simulink model "traffic"  (R2017a)
settings: Solver=ode45  StartTime=0.0  StopTime=30.0  RelTol=1e-3  EnableMultiTasking=on
undefined symbols (not defined in the file): des, gcbh
settings Model: Creator=pathmapirian  LastModifiedBy=PRAGA SV
settings DataIOCC: LimitDataPoints=on  SaveFormat=Array
settings OptimizationCC: LifeSpan=inf
settings DebuggingCC: UnderspecifiedInitializationDetection=Classic  MergeDetectMultiDrivingBlocksExec=none  SolverPrmCheckMsg=warning  StateNameClashWarn=warning  SFUnexpectedBacktrackingDiag=warning  SFNoUnconditionalDefaultTransitionDiag=warning  SFExecutionAtInitializationDiag=none
settings HardwareCC: ProdBitPerPointer=32  ProdBitPerSizeT=32  ProdBitPerPtrDiffT=32  ProdLargestAtomicFloat=None  ProdIntDivRoundTo=Undefined  ProdEndianess=Unspecified  ProdWordSize=32  ProdHWDeviceType=32-bit Generic
settings ModelReferenceCC: PropagateSignalLabelsOutOfModel=off
settings GRTTargetCC: TargetLangStandard=C89/C90 (ANSI)  GeneratePreprocessorConditionals=Disable all
settings ConfigComp: CovMetricSettings=dw  CovHtmlReporting=on  CovSaveCumulativeToWorkspaceVar=on  CovSaveSingleToWorkspaceVar=on  CovExternalEMLEnable=off

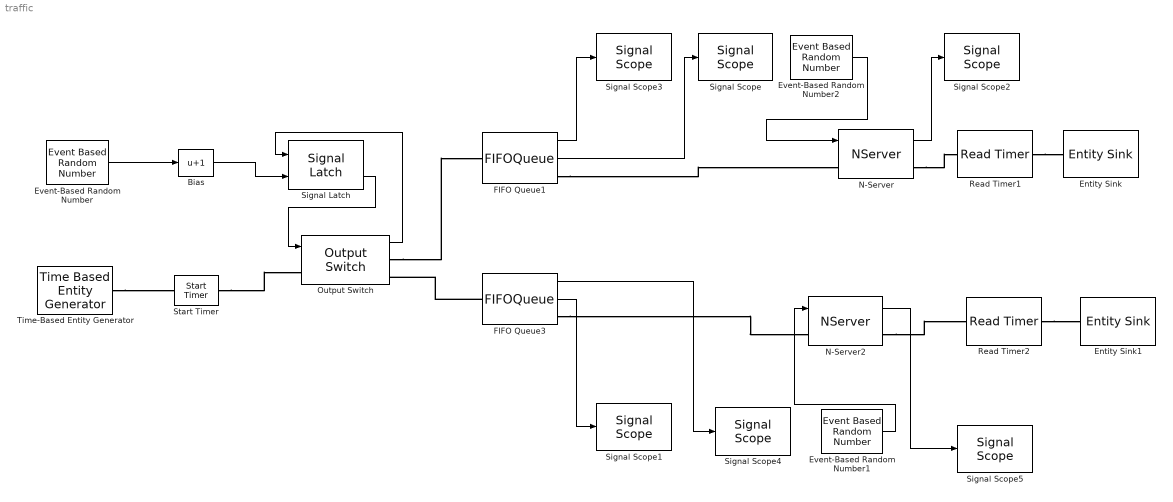
== system traffic ==
  Bias : Bias  Bias=1
  Entity Sink : EntitySink
  Entity Sink1 : EntitySink
  Event-Based Random Number : EventBasedRandomNumber  Distribution=Bernoulli  pOneBern=0.6  Seed=10
  Event-Based Random Number1 : EventBasedRandomNumber  Distribution=Uniform
  Event-Based Random Number2 : EventBasedRandomNumber
  FIFO Queue1 : FIFOQueue  StatNumberInBlock=on  StatAverageWait=on
      settings: OutputPortMap=o1,o2
  FIFO Queue3 : FIFOQueue  StatNumberInBlock=on  StatAverageWait=on
      settings: OutputPortMap=o1,o2
  N-Server : NServer  NumberOfServers=1  ServiceTimeFrom=Signal port t  StatUtilization=on
      settings: OutputPortMap=o5
  N-Server2 : NServer  NumberOfServers=1  ServiceTimeFrom=Signal port t  StatUtilization=on
      settings: OutputPortMap=o5
  Output Switch : OutputSwitch  NumberOutputPorts=2  SwitchingCriterion=From signal port p  InitialConditionsOpt=on  StatNumberDeparted=on
  Read Timer1 : ReadTimer
  Read Timer2 : ReadTimer
  Signal Latch : SignalLatch  ReadMemoryUpon=Write to memory event  ReportMemoryUponWrite=on
      settings: InputPortMap=u0,u2  OutputPortMap=o1,o2
  Signal Scope{,1..5} (6 alike) : SignalScope  LoadFcn=des.scope.CallbackSupport('seLoadFcn',gcbh)  StartFcn=des.scope.CallbackSupport('seStartFcn',gcbh)  StopFcn=des.scope.CallbackSupport('seStopFcn',gcbh)
      settings: CopyFcn=des.scope.CallbackSupport('seCopyFcn',gcbh)  DeleteFcn=des.scope.CallbackSupport('seDeleteFcn',gcbh)  PreSaveFcn=des.scope.CallbackSupport('sePreSaveFcn',gcbh)  NameChangeFcn=des.scope.CallbackSupport('seNameChangeFcn',gcbh)  OpenFcn=des.scope.CallbackSupport('seOpenFcn',gcbh)
  Start Timer : StartTimer
  Time-Based Entity Generator : TimeBasedEntityGenerator
  wires:
  FIFO Queue1/1 -> Signal Scope3/1
  FIFO Queue1/2 -> Signal Scope/1
  Event-Based Random Number2/1 -> N-Server/1
  N-Server/1 -> Signal Scope2/1
  FIFO Queue3/2 -> Signal Scope1/1
  FIFO Queue3/1 -> Signal Scope4/1
  Event-Based Random Number1/1 -> N-Server2/1
  N-Server2/1 -> Signal Scope5/1
  Event-Based Random Number/1 -> Bias/1
  Bias/1 -> Signal Latch/2
  Output Switch/1 -> Signal Latch/1
  Signal Latch/2 -> Output Switch/1
  connections:
  Time-Based Entity Generator/RConn1 -- Start Timer/LConn1
  Start Timer/RConn1 -- Output Switch/LConn1
  Output Switch/RConn1 -- FIFO Queue1/LConn1
  FIFO Queue3/LConn1 -- Output Switch/RConn2
  FIFO Queue1/RConn1 -- N-Server/LConn1
  N-Server/RConn1 -- Read Timer1/LConn1
  FIFO Queue3/RConn1 -- N-Server2/LConn1
  N-Server2/RConn1 -- Read Timer2/LConn1
  Read Timer1/RConn1 -- Entity Sink/LConn1
  Read Timer2/RConn1 -- Entity Sink1/LConn1
